simulink model "My_NSS_Model"  (R2026a)
settings: Solver=VariableStepAuto
libraries: slident x1

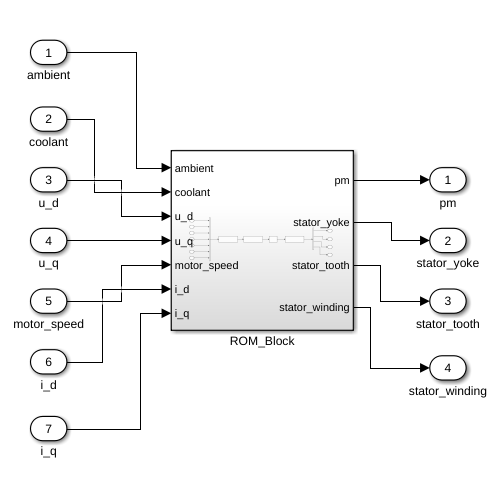
[thumbnail: Simulink's stored preview of the top-level diagram]
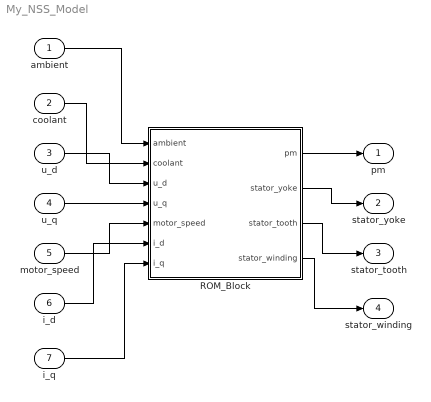
== system My_NSS_Model ==
  ambient : Inport
  coolant : Inport  Port=2
  u_d : Inport  Port=3
  u_q : Inport  Port=4
  motor_speed : Inport  Port=5
  i_d : Inport  Port=6
  i_q : Inport  Port=7
  ROM_Block : Subsystem  Description=This block requires workspace variable NSSModel loaded from /MATLAB Drive/ROM Workshop/02a-ROM of a PMSM Motor/ROM_PMSM_ExperimentManager/NSS_ExperimentProject/trainingOutput.mat.
  pm : Outport
  stator_yoke : Outport  Port=2
  stator_tooth : Outport  Port=3
  stator_winding : Outport  Port=4
  wires:
  ROM_Block/3(stator_tooth) -> stator_tooth/1
  ROM_Block/1(pm) -> pm/1
  i_q/1 -> ROM_Block/7(i_q)
  i_d/1 -> ROM_Block/6(i_d)
  motor_speed/1 -> ROM_Block/5(motor_speed)
  ROM_Block/2(stator_yoke) -> stator_yoke/1
  u_q/1 -> ROM_Block/4(u_q)
  ROM_Block/4(stator_winding) -> stator_winding/1
  u_d/1 -> ROM_Block/3(u_d)
  coolant/1 -> ROM_Block/2(coolant)
  ambient/1 -> ROM_Block/1(ambient)

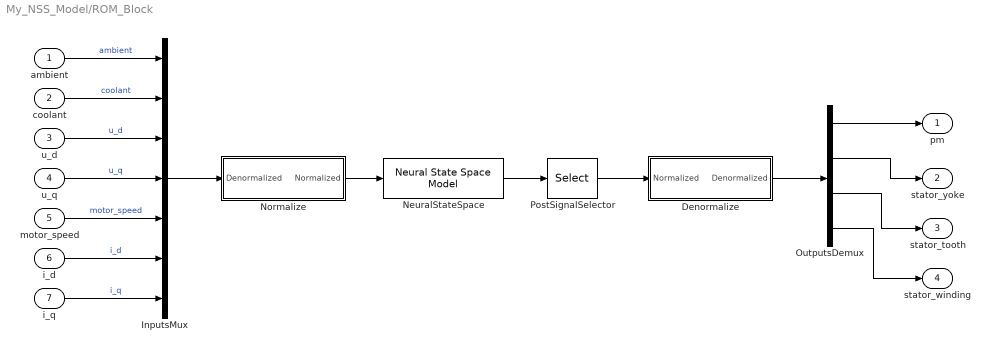
== system My_NSS_Model/ROM_Block ==
  ambient : Inport
  coolant : Inport  Port=2
  u_d : Inport  Port=3
  u_q : Inport  Port=4
  motor_speed : Inport  Port=5
  i_d : Inport  Port=6
  i_q : Inport  Port=7
  Denormalize : Subsystem
      mask Display: disp('Denormalize')
  InputsMux : Mux  Inputs=7
  NeuralStateSpace : slident/Models/Neural State Space Model  sys=NSSModel  x0type=internal  ic=0  returnx=off  returndx=off
  Normalize : Subsystem
      mask Display: disp('Normalize')
  OutputsDemux : Demux
  PostSignalSelector : Selector  InputPortWidth=4  IndexOptions=Index vector (dialog)  Indices=[1;2;3;4]  OutputSizes=1
  pm : Outport
  stator_yoke : Outport  Port=2
  stator_tooth : Outport  Port=3
  stator_winding : Outport  Port=4
  wires:
  OutputsDemux/3 -> stator_tooth/1
  OutputsDemux/2 -> stator_yoke/1
  ambient/1 -> InputsMux/1  "ambient"
  OutputsDemux/4 -> stator_winding/1
  u_d/1 -> InputsMux/3  "u_d"
  u_q/1 -> InputsMux/4  "u_q"
  motor_speed/1 -> InputsMux/5  "motor_speed"
  NeuralStateSpace/1 -> PostSignalSelector/1
  InputsMux/1 -> Normalize/1(Denormalized)
  i_q/1 -> InputsMux/7  "i_q"
  Normalize/1(Normalized) -> NeuralStateSpace/1
  i_d/1 -> InputsMux/6  "i_d"
  PostSignalSelector/1 -> Denormalize/1(Normalized)
  coolant/1 -> InputsMux/2  "coolant"
  Denormalize/1(Denormalized) -> OutputsDemux/1
  OutputsDemux/1 -> pm/1

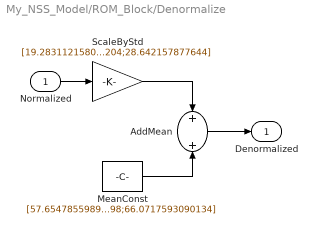
== system My_NSS_Model/ROM_Block/Denormalize ==
  Normalized : Inport
  AddMean : Sum
  MeanConst : Constant  Value=[57.6547855989914;47.7434565483279;56.4769677508298;66.0717593090134]
  ScaleByStd : Gain  Gain=[19.2831121580692;19.768310013522;22.8933717955204;28.642157877644]
  Denormalized : Outport
  wires:
  AddMean/1 -> Denormalized/1
  MeanConst/1 -> AddMean/2
  ScaleByStd/1 -> AddMean/1
  Normalized/1 -> ScaleByStd/1

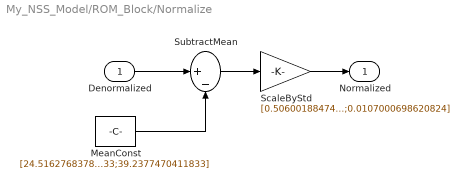
== system My_NSS_Model/ROM_Block/Normalize ==
  Denormalized : Inport
  MeanConst : Constant  Value=[24.516276837834;35.6640979220904;-24.9932014089761;54.6611484273913;2214.0987153129;-69.5447341480833;39.2377470411833]
  ScaleByStd : Gain  Gain=[0.506001884749666;0.0471536510398972;0.0160495479762288;0.0223153352616547;0.000531907245665926;0.0156440002950235;0.0107000698620824]
  SubtractMean : Sum  Inputs=|+-
  Normalized : Outport
  wires:
  SubtractMean/1 -> ScaleByStd/1
  MeanConst/1 -> SubtractMean/2
  ScaleByStd/1 -> Normalized/1
  Denormalized/1 -> SubtractMean/1
